simulink model "GFM_cir_exp"  (R2025a)
settings: Solver=FixedStepAuto  StartTime=0.0  StopTime=t_end+t_sim_start  FixedStep=Ts  RelTol=1e-3
InitFcn:
  | run GFMPara_exp.m
values from neighbouring files (symbols this model uses):
  Cf = 0.0083    [GFMPara.m]    (also in GFMPara_exp.m = 0.0249; VFMPara.m = 0.02; VFMPara_exp.m = 0.03)
  dt_sag = t_c    [GFMPara.m]    (also in GFMPara_exp.m; PLLpara.m; VFMPara.m; VFMPara_exp.m)
  f_switching = 20e3    (= 20000)    [GFMPara_exp.m]    (also in PLLpara.m = 10000; VFMPara_exp.m)
  Lc = 1e-9    (= 1e-09)    [GFMPara.m]    (also in GFMPara_exp.m; PLLpara.m; VFMPara.m; VFMPara_exp.m)
  Lf = 0.0592    [GFMPara.m]    (also in GFMPara_exp.m; PLLpara.m = 0.05; VFMPara.m = 0.05; VFMPara_exp.m = 0.05)
  m_gfm = 1/D    [GFMPara.m]    (also in GFMPara_exp.m)
  Pm = Pm    [GFMPara.m]    (also in GFMPara_exp.m)
  Sbase = 1    [GFMPara.m]    (also in GFMPara_exp.m; PLLpara.m; VFMPara.m; VFMPara_exp.m)
  Scale_ki_v = 20    [GFMPara.m]    (also in GFMPara_exp.m; VFMPara.m; VFMPara_exp.m)
  t0_sag = t_sim_start +t_start    [GFMPara.m]    (also in GFMPara_exp.m; PLLpara.m = 20; VFMPara.m; VFMPara_exp.m = 20)
  Tc = 1/f_switching    (= 5e-05)    [GFMPara_exp.m]    (also in PLLpara.m = 0.0001; VFMPara_exp.m)
  Ts = 1/Fs    (= 1e-05)    [GFMPara.m]    (also in GFMPara_exp.m = 1e-06; PLLpara.m = 1e-06; VFMPara.m = 5e-06; VFMPara_exp.m = 1e-06)
  v_sag = Ug_fault    [GFMPara.m]    (also in GFMPara_exp.m; PLLpara.m; VFMPara.m; VFMPara_exp.m)
  Vbase = 1    [GFMPara.m]    (also in GFMPara_exp.m; PLLpara.m; VFMPara.m; VFMPara_exp.m)
  Vdc_ref = 2.5    [GFMPara_exp.m]
  w_droop = D/J    [GFMPara.m]    (also in GFMPara_exp.m; VFMPara.m = 314.159265359; VFMPara_exp.m = 314.159265359)
  w_i_GFM = 2000*2*pi    (= 12566.3706144)    [GFMPara.m]    (also in GFMPara_exp.m = 9424.77796077; VFMPara.m = 9424.77796077; VFMPara_exp.m = 9424.77796077)
  w_v_GFM = 800 *2*pi    (= 5026.54824574)    [GFMPara.m]    (also in GFMPara_exp.m = 3141.59265359; VFMPara.m = 3141.59265359; VFMPara_exp.m = 3141.59265359)
  Wbase = 2*pi*50    (= 314.159265359)    [GFMPara.m]    (also in GFMPara_exp.m; PLLpara.m; VFMPara.m; VFMPara_exp.m)
  Zbase = Vbase/Ibase    (= 1)    [GFMPara.m]    (also in GFMPara_exp.m; PLLpara.m; VFMPara.m; VFMPara_exp.m)
undefined symbols (not defined in the file or in its folder): D, DiscIntNeverNeededParam, dspblkCoreblockFVToolHelper, gcbh, Ilim, initial, J, Rg, Xg, Y_dc
libraries: spsVoltageMeasurementLib x31, spsCurrentMeasurementLib x30, spsControlledVoltageSourceLib x9, spsThreePhaseSeriesRLCBranchLib x8, spsSeriesRLCBranchLib x7, spsHalfBridgeConverterLib x3, spsDCVoltageSourceLib x1, simulink x1, spspowerguiLib x1
(part 3 of 3)

== system GFM_cir_exp/Grid-Forming Inverter (Simulink Block)1/Voltage Controller/Circular Current Limiter ==
  note: Hard circular current limiter: rho = min(1, Imax/||i_raw||), i_lim = rho*i_raw.
      | The mismatch delta_i = i_raw-i_lim is returned for anti-windup feedback.
  i_raw_dq : Inport  SampleTime=Tc
  Anti-windup z^-1 : UnitDelay  SampleTime=Ts
  Compare To Constant : simulink/Logic and Bit Operations/Compare To Constant  relop=<  const=Imax  OutDataTypeStr=boolean
  Complex to Magnitude-Angle : ComplexToMagnitudeAngle
  Complex to Real-Imag : ComplexToRealImag
  Data Type Conversion : DataTypeConversion  OutDataTypeStr=double  SaturateOnIntegerOverflow=off  RndMeth=Floor
  Magnitude-Angle to Complex : MagnitudeAngleToComplex
  Mux : Mux  Inputs=2
  Mux1 : Mux  Inputs=2
  Real-Imag to Complex : RealImagToComplex
  Scope : Scope
      settings: ActiveDisplayYMinimum=1.3254699767797136  ActiveDisplayYMaximum=1.7812555131289503  DataLoggingVariableName=ScopeData14
  Scope1 : Scope
      settings: ActiveDisplayYMinimum=-0.12499999999999997  ActiveDisplayYMaximum=1.125  DataLoggingVariableName=ScopeData16
  Scope2 : Scope
      settings: ActiveDisplayYMinimum=-0.061758895540843767  ActiveDisplayYMaximum=0.084269010178629783  DataLoggingVariableName=ScopeData17
  delta_i = i_raw-i_lim : Sum  Inputs=+-
  dq : Demux  Outputs=2
  rho = min(1,Imax divided by magnitude) : Saturate  UpperLimit=Imax  LowerLimit=0
  i_lim_dq : Outport
  delta_i_dq : Outport  Port=2
  lim_en : Outport  Port=3
  wires:
  i_raw_dq/1 -> dq/1, delta_i = i_raw-i_lim/1
  Real-Imag to Complex/1 -> Complex to Magnitude-Angle/1
  dq/1 -> Real-Imag to Complex/1
  dq/2 -> Real-Imag to Complex/2
  rho = min(1,Imax divided by magnitude)/1 -> Mux1/2, Magnitude-Angle to Complex/1
  Compare To Constant/1 -> Data Type Conversion/1
  Data Type Conversion/1 -> Anti-windup z^-1/1
  Complex to Magnitude-Angle/1 -> rho = min(1,Imax divided by magnitude)/1, Mux1/1, Compare To Constant/1
  Complex to Magnitude-Angle/2 -> Magnitude-Angle to Complex/2
  Magnitude-Angle to Complex/1 -> Complex to Real-Imag/1
  Complex to Real-Imag/2 -> Mux/2
  Complex to Real-Imag/1 -> Mux/1
  Mux/1 -> delta_i = i_raw-i_lim/2, i_lim_dq/1
  Mux1/1 -> Scope/1
  Anti-windup z^-1/1 -> Scope1/1, lim_en/1
  delta_i = i_raw-i_lim/1 -> Scope2/1, delta_i_dq/1

== system GFM_cir_exp/Grid-Forming Inverter (Simulink Block)1/Voltage Controller/PI-DT-Estimated d ==
  enable : Inport
  reference : Inport  Port=2
  initial : Inport  Port=3
  actual : Inport  Port=4
  Int_en : Inport  Port=5
  Discrete-Time Integrator : DiscreteIntegrator  gainval=1  ExternalReset=rising  InitialConditionSource=external  InitialCondition=initial  SampleTime=Ts  LimitOutput=on  UpperSaturationLimit=xmax  LowerSaturationLimit=xmin  ICPrevOutput=DiscIntNeverNeededParam  ICPrevScaledInput=DiscIntNeverNeededParam
  Ierror : Sum  Inputs=+-
  Ki : Gain  Gain=Ki  SaturateOnIntegerOverflow=on  OutDataTypeStr=Inherit: Same as input  ParamDataTypeStr=Inherit: Same as input
  Kp : Gain  Gain=Kp  SaturateOnIntegerOverflow=on  OutDataTypeStr=Inherit: Same as input  ParamDataTypeStr=Inherit: Same as input
  Perror : Sum  Inputs=-+
  Product{,1..3} (4 alike) : Product  RndMeth=Zero
  Saturation : Saturate  UpperLimit=xmax  LowerLimit=xmin
  Scope : Scope
      settings: ActiveDisplayYMinimum=0.10946560967336291  ActiveDisplayYMaximum=0.2336316811358759  DataLoggingVariableName=ScopeData4
  Scope1 : Scope
      settings: ActiveDisplayYMinimum=-0.536169938501879  ActiveDisplayYMaximum=1.1699196606068656  DataLoggingVariableName=ScopeData11
  Sum1 : Sum  SaturateOnIntegerOverflow=on
  Out : Outport
  wires:
  Ierror/1 -> Product1/1
  Product/1 -> Kp/1
  Perror/1 -> Scope1/1, Product/1
  reference/1 -> Ierror/1, Perror/2
  actual/1 -> Ierror/2, Perror/1
  initial/1 -> Discrete-Time Integrator/3
  enable/1 -> Product1/2, Product/2, Product2/1
  Kp/1 -> Sum1/1
  Ki/1 -> Discrete-Time Integrator/1
  Sum1/1 -> Saturation/1
  Saturation/1 -> Out/1
  Int_en/1 -> Product2/2
  Product2/1 -> Product3/2, Discrete-Time Integrator/2
  Discrete-Time Integrator/1 -> Product3/1
  Product3/1 -> Scope/1, Sum1/2
  Product1/1 -> Ki/1

== system GFM_cir_exp/Grid-Forming Inverter (Simulink Block)1/Voltage Controller/PI-DT-Estimated q ==
  actual : Inport
  initial : Inport  Port=2
  reference : Inport  Port=3
  enable : Inport  Port=4
  Int_en : Inport  Port=5
  Discrete-Time Integrator : DiscreteIntegrator  gainval=1  ExternalReset=rising  InitialConditionSource=external  InitialCondition=initial  SampleTime=Ts  LimitOutput=on  UpperSaturationLimit=xmax  LowerSaturationLimit=xmin  ICPrevOutput=DiscIntNeverNeededParam  ICPrevScaledInput=DiscIntNeverNeededParam
  Ierror : Sum  Inputs=+-
  Ki : Gain  Gain=Ki  SaturateOnIntegerOverflow=on  OutDataTypeStr=Inherit: Same as input  ParamDataTypeStr=Inherit: Same as input
  Kp : Gain  Gain=Kp  SaturateOnIntegerOverflow=on  OutDataTypeStr=Inherit: Same as input  ParamDataTypeStr=Inherit: Same as input
  Perror : Sum  Inputs=-+
  Product{,1..3} (4 alike) : Product  RndMeth=Zero
  Saturation : Saturate  UpperLimit=xmax  LowerLimit=xmin
  Scope : Scope
      settings: ActiveDisplayYMinimum=-0.0046770125700697366  ActiveDisplayYMaximum=0.014647816665555792  DataLoggingVariableName=ScopeData8
  Scope1 : Scope
      settings: ActiveDisplayYMinimum=-0.15120291351856477  ActiveDisplayYMaximum=0.43649131539385444  DataLoggingVariableName=ScopeData12
  Scope2 : Scope
      settings: ActiveDisplayYMinimum=-0.60333298312215922  ActiveDisplayYMaximum=0.001341350170408373  DataLoggingVariableName=ScopeData18
  Sum1 : Sum  SaturateOnIntegerOverflow=on
  Out : Outport
  wires:
  Ierror/1 -> Product1/1
  Product/1 -> Kp/1
  Perror/1 -> Scope1/1, Product/1
  reference/1 -> Ierror/1, Perror/2
  actual/1 -> Perror/1, Ierror/2
  initial/1 -> Discrete-Time Integrator/3, Scope2/1
  enable/1 -> Product2/1, Product1/2, Product/2
  Kp/1 -> Sum1/1
  Ki/1 -> Discrete-Time Integrator/1
  Sum1/1 -> Saturation/1
  Saturation/1 -> Out/1
  Int_en/1 -> Product2/2
  Discrete-Time Integrator/1 -> Product3/1
  Product3/1 -> Sum1/2, Scope/1
  Product1/1 -> Ki/1
  Product2/1 -> Product3/2, Discrete-Time Integrator/2

== system GFM_cir_exp/Grid-Forming Inverter (Simulink Block)1/modulator/Triangle ==
  Constant1 : Constant  Value=0.5
  Constant2 : Constant  Value=-pi/2
  Constant4 : Constant  Value=2*pi
  Freq1 : Constant  Value=f_switching
  Freq2 : Constant  Value=2*pi
  Gain1 : Gain  Gain=1/pi  SaturateOnIntegerOverflow=on  OutDataTypeStr=Inherit: Same as input  ParamDataTypeStr=Inherit: Same as input
  Math Function : Math  Operator=mod  SignedPower=on
  Product : Product  Inputs=***  InputSameDT=on  SaturateOnIntegerOverflow=on  OutDataTypeStr=Inherit: Same as first input
  Scope1 : Scope
      settings: ActiveDisplayYMinimum=-0.099307460614389  ActiveDisplayYMaximum=1.0691420983565338  DataLoggingVariableName=ScopeData19
  Sum : Sum  InputSameDT=on  SaturateOnIntegerOverflow=on  OutDataTypeStr=Inherit: Same as first input
  Sum1 : Sum  InputSameDT=on  SaturateOnIntegerOverflow=on  OutDataTypeStr=Inherit: Same as first input
  Trigonometric Function : Trigonometry  Operator=asin
  Trigonometric Function3 : Trigonometry
  t : DigitalClock  SampleTime=Ts
  carrier_wav : Outport
  wires:
  Trigonometric Function3/1 -> Trigonometric Function/1
  Trigonometric Function/1 -> Gain1/1
  Math Function/1 -> Trigonometric Function3/1
  Constant4/1 -> Math Function/2
  Freq1/1 -> Product/1
  Freq2/1 -> Product/3
  t/1 -> Product/2
  Gain1/1 -> Sum1/1
  Sum1/1 -> Scope1/1, carrier_wav/1
  Constant1/1 -> Sum1/2
  Product/1 -> Sum/1
  Sum/1 -> Math Function/1
  Constant2/1 -> Sum/2
